simulink model "Exercise11_1"  (R2018b)
settings: Solver=VariableStepAuto  StartTime=0.0  StopTime=10.0  RelTol=1e-3
settings Model: Creator=Ramiro  LastModifiedBy=Ramiro

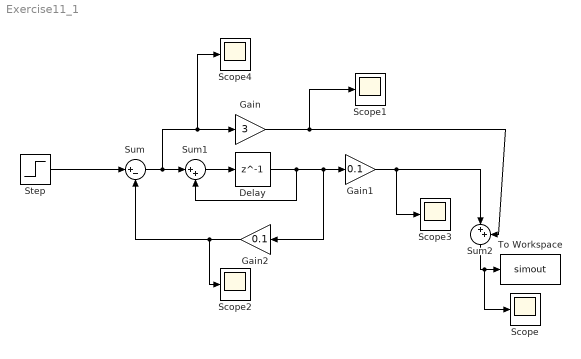
== system Exercise11_1 ==
  Delay : Delay  DelayLength=1  InitialCondition=0
  Gain : Gain  Gain=3
  Gain1 : Gain  Gain=0.1
  Gain2 : Gain  Gain=0.1
  Scope{,1..4} (5 alike) : Scope
  Step : Step  SampleTime=0
  Sum : Sum  Inputs=|+-
  Sum1 : Sum  Inputs=|++
  Sum2 : Sum  Inputs=|++
  To Workspace : ToWorkspace  VariableName=simout  SaveFormat=Timeseries  SampleTime=-1
  wires:
  Step/1 -> Sum/1
  Sum1/1 -> Delay/1
  Sum/1 -> Scope4/1, Gain/1, Sum1/1
  Delay/1 -> Sum1/2, Gain2/1, Gain1/1
  Gain1/1 -> Scope3/1, Sum2/1
  Gain/1 -> Scope1/1, Sum2/2
  Gain2/1 -> Scope2/1, Sum/2
  Sum2/1 -> Scope/1, To Workspace/1
